simulink model "GenericMotorModel"  (R2023a)
settings: Solver=VariableStepAuto  StartTime=0.0  StopTime=10.0  RelTol=1e-3
values from neighbouring files (symbols this model uses):
  J = zeros(1, iters)    [ift.m]
undefined symbols (not defined in the file or in its folder): B, Km, Rw
settings Model: Creator=bl4ck  LastModifiedBy=bl4ck

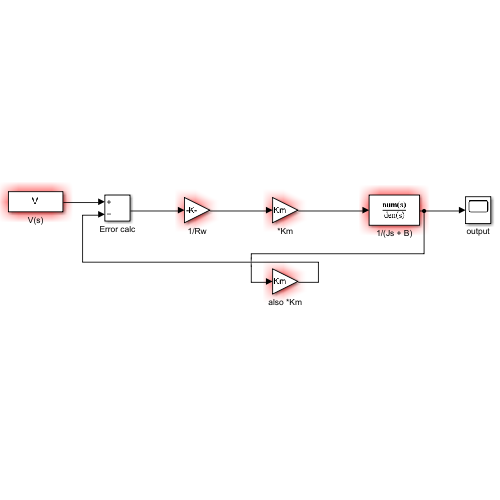
[thumbnail: Simulink's stored preview of the top-level diagram]
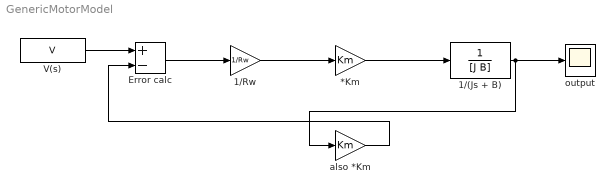
== system GenericMotorModel ==
  *Km : Gain  Gain=Km
  1/(Js + B) : TransferFcn  Denominator=[J B]
  1/Rw : Gain  Gain=1/Rw
  Error calc : Sum  Inputs=+-
  V(s) : FromWorkspace  VariableName=V
  also *Km : Gain  Gain=Km
  output : Scope
  wires:
  V(s)/1 -> Error calc/1
  Error calc/1 -> 1/Rw/1
  1/Rw/1 -> *Km/1
  *Km/1 -> 1/(Js + B)/1
  1/(Js + B)/1 -> also *Km/1, output/1
  also *Km/1 -> Error calc/2
